simulink model "First_Simulation_file"  (R2017b)
settings: Solver=VariableStepAuto  StartTime=0.0  StopTime=10.0  RelTol=1e-3
settings Model: Creator=Obriel  LastModifiedBy=Obriel

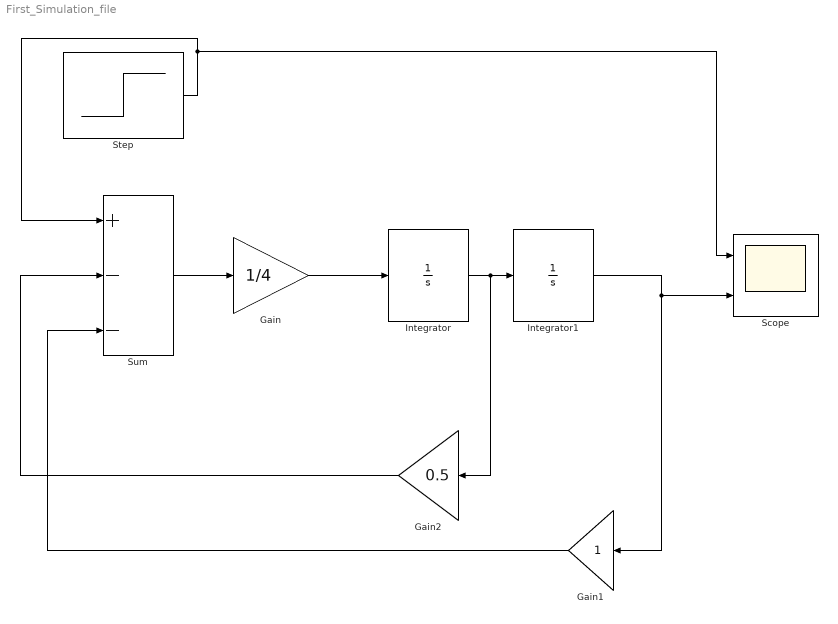
== system First_Simulation_file ==
  Gain : Gain  Gain=1/4
  Gain1 : Gain
  Gain2 : Gain  Gain=0.5
  Integrator : Integrator
  Integrator1 : Integrator
  Scope : Scope  NumInputPorts=2
  Step : Step  Time=3  After=3  SampleTime=0
  Sum : Sum  Inputs=+--
  wires:
  Sum/1 -> Gain/1
  Gain/1 -> Integrator/1
  Integrator/1 -> Gain2/1, Integrator1/1
  Integrator1/1 -> Scope/2, Gain1/1
  Gain2/1 -> Sum/2
  Gain1/1 -> Sum/3
  Step/1 -> Scope/1, Sum/1
